simulink model "ProModel"  (R2024b)
settings: Solver=VariableStepAuto  StartTime=0.0  StopTime=10.0  MaxStep=5  RelTol=1e-3
values from neighbouring files (symbols this model uses):
  Cvg = cpo*roo*Vg    (= 182424.96)    [Lab1.m]
  Cvw = cpp*rop*Vw    (= 105000)    [Lab1.m]
  dPg = 0    [Lab1.m]    (also in Lab1cz2.m)
  dTzew = 1    [Lab1.m]    (also in Lab1cz2.m)
  K1 = K12/2    (= 25)    [Lab1.m]    (also in Lab1cz2.m)
  K2 = K12/2    (= 25)    [Lab1.m]    (also in Lab1cz2.m)
  Kg = PgN/(TgN-TwewN)    (= 100)    [Lab1.m]    (also in Lab1cz2.m)
  Pg0 = tab_Pg(i)    [Lab1.m]    (also in Lab1cz2.m)
  Tg0 = (Pg0+Kg*Twew0)/Kg    [Lab1.m]    (also in Lab1cz2.m = x(1))
  Twew0 = (Pg0+(K1+K2)*Tzew0)/(K1+K2)    [Lab1.m]    (also in Lab1cz2.m = x(2))
  Tzew0 = tab_Tzew(i)    [Lab1.m]    (also in Lab1cz2.m)
settings Model: Creator=konradlandzberg  LastModifiedBy=konradlandzberg

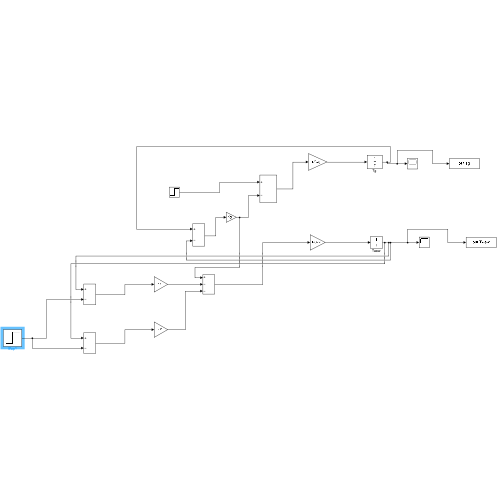
[thumbnail: Simulink's stored preview of the top-level diagram]
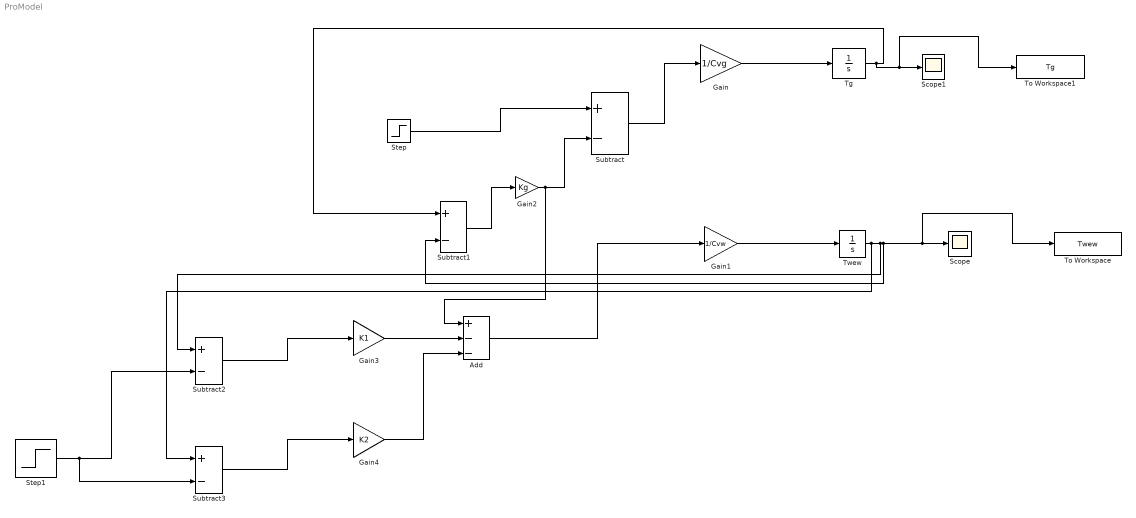
== system ProModel ==
  Add : Sum  Inputs=+--
  Gain : Gain  Gain=1/Cvg
  Gain1 : Gain  Gain=1/Cvw
  Gain2 : Gain  Gain=Kg
  Gain3 : Gain  Gain=K1
  Gain4 : Gain  Gain=K2
  Scope : Scope
  Scope1 : Scope
  Step : Step  Time=5000  Before=Pg0  After=Pg0+dPg  SampleTime=0
  Step1 : Step  Time=5000  Before=Tzew0  After=Tzew0+dTzew  SampleTime=0
  Subtract{,1..3} (4 alike) : Sum  Inputs=+-
  Tg : Integrator  InitialCondition=Tg0
  To Workspace : ToWorkspace  VariableName=Twew  SampleTime=-1
  To Workspace1 : ToWorkspace  VariableName=Tg  SampleTime=-1
  Twew : Integrator  InitialCondition=Twew0
  wires:
  Gain/1 -> Tg/1
  Gain1/1 -> Twew/1
  Subtract/1 -> Gain/1
  Step/1 -> Subtract/1
  Gain2/1 -> Add/1, Subtract/2
  Subtract1/1 -> Gain2/1
  Twew/1 -> Subtract3/1, Subtract2/1, Subtract1/2, To Workspace/1, Scope/1
  Tg/1 -> To Workspace1/1, Scope1/1, Subtract1/1
  Add/1 -> Gain1/1
  Gain3/1 -> Add/2
  Gain4/1 -> Add/3
  Subtract3/1 -> Gain4/1
  Subtract2/1 -> Gain3/1
  Step1/1 -> Subtract3/2, Subtract2/2
